simulink model "control_sys_hardware"  (R2024b)
settings: Solver=ode5  StartTime=0.0  StopTime=inf  FixedStep=.0005  RelTol=1e-3
values from neighbouring files (symbols this model uses):
  A = [0, 1, 0, 0, 0, 0, 0, 0, 0 ... (first row only)    [control_sys.m]
  B = [0, 0, 0 ... (first row only)    [control_sys.m]
  b_eq_phi = (n^2)*b_r1 + b_r2 + b_load_phi    (= 46.8203648256)    [control_sys.m]
  b_eq_r = 0.06    [control_sys.m]
  b_eq_theta = (n^2)*b_r1 + b_r2 + b_load_theta    (= 46.8203648256)    [control_sys.m]
  C = [1 0 0 0 0 0 0 0 0 ... (first row only)    [control_sys.m]
  D = [0 0 0 ... (first row only)    [control_sys.m]
  g = 9.81    [control_sys.m]
  J_act_const_phi = (J_act_vert + J_act_horiz)/2    (= 0.17578)    [control_sys.m]
  J_act_const_theta = ((m_act_base + m_act_case + m_act_screw)*(.5588^2) + m_act_rod*(.508^2))/3    (= 0.139191119467)    [control_sys.m]
  J_act_var_phi = (J_act_vert - J_act_horiz)/2    (= -0.17078)    [control_sys.m]
  J_const_phi = J_m1out + J_load_phi    (= 101.81800125)    [control_sys.m]
  J_const_theta = J_m2out    (= 102.01900125)    [control_sys.m]
  J_eq_r = 0.0018    [control_sys.m]
  K = lqr(A,B,Q,R)    [control_sys.m]
  K_r1 = .11    (= 0.11)    [control_sys.m]
  K_r2 = .11    (= 0.11)    [control_sys.m]
  K_r3 = 0.0709    [control_sys.m]
  Kr = inv(C*inv(-A+B*K)*B)    [control_sys.m]
  L_a1 = 0.3    [control_sys.m]
  L_a2 = 0.3    [control_sys.m]
  L_a3 = 0.09    [control_sys.m]
  l_act_const = 0.550    (= 0.55)    [control_sys.m]
  l_act_rod = 0.511175    [control_sys.m]
  m_act = m_act_base + m_act_rod + m_act_screw + m_act_case + m_load    (= 1.364)    [control_sys.m]
  m_act_rod = 0.154    [control_sys.m]
  m_load = 0    [control_sys.m]
  n = 184    [control_sys.m]
  n_3 = 3.07500    (= 3.075)    [control_sys.m]
  p_s = 0.0035    [control_sys.m]
  R_a1 = 1.36    [control_sys.m]
  R_a2 = 1.36    [control_sys.m]
  R_a3 = 2.0500    (= 2.05)    [control_sys.m]
  r_cg_const = (l_act_const*.5*(m_act_case + m_act_screw) + .06*m_act_base)/m_act    (= 0.150795454545)    [control_sys.m]
  tomato_positions = [34; 60; 12.5]    [control_sys.m]
undefined symbols (not defined in the file or in its folder): Continuous, National_Instruments, PCIe, Time
libraries: simulink x15, spsEdgeDetectorLib x15, sldrtlib x13, ctrlSharedLib x1
settings Model: SimulationMode=external  Creator=jcglenn  LastModifiedBy=jcglenn
settings DebuggingCC: UnderSpecifiedDimensionMsg=warning
settings HardwareCC: ProdBitPerLong=64  ProdHWDeviceType=Intel->x86-64 (Linux 64)
settings RTWCC: Description=Simulink Desktop Real-Time  SystemTargetFile=sldrt.tlc  TemplateMakefile=sldrt.tmf  RTWCompilerOptimization=on
settings CodeAppCC: MaxIdLength=95
settings SimulinkDesktopRealTimeCC: TargetLibSuffix=_sldrt.a  TargetPreCompLibLocation=C:\Program Files\MATLAB\R2024b\toolbox\sldrt\lib\win64  ParMdlRefBuildCompliant=on

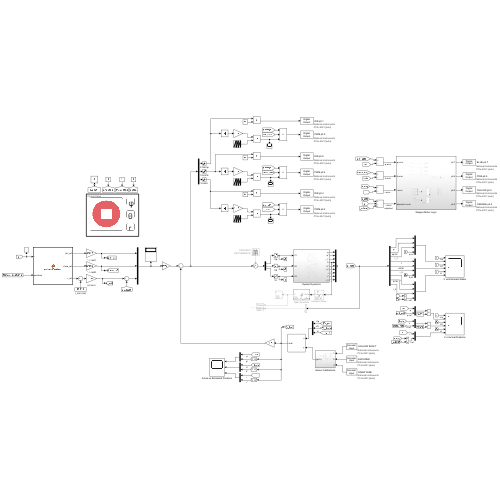
[thumbnail: Simulink's stored preview of the top-level diagram]
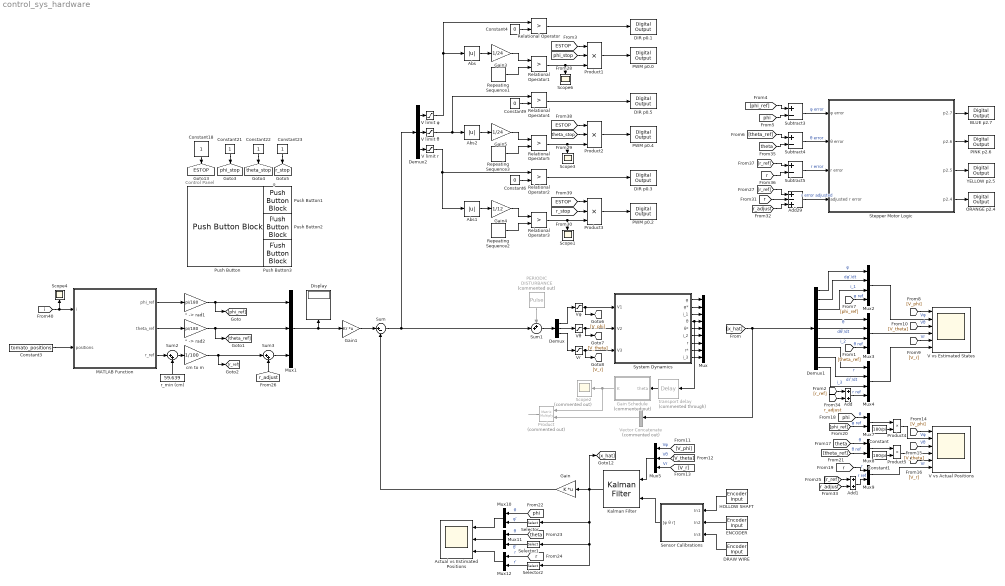
== system control_sys_hardware ==
  note: Control Panel
  note: φ
  note: θ
  note: r
  Abs : Abs  SaturateOnIntegerOverflow=off
  Abs1 : Abs  SaturateOnIntegerOverflow=off
  Abs2 : Abs  SaturateOnIntegerOverflow=off
  Actual vs Estimated Positions : Scope  NumInputPorts=3
  Add : Sum
  Add1 : Sum
  Add29 : Sum  Inputs=+-+
  BLUE p2.7 : sldrtlib/Digital Output  SampleTime=.001  MaxMissedTicks=100  ShowMissedTicks=off  YieldWhenWaiting=off  DrvName=National_Instruments/PCIe-6321  DrvAddress=4294967295  DrvOptions=[0 3 61440 2 0 0 0]  Channels=48  BitMode=1  InitialValue=[]  FinalValue=[]
      settings: AttributesFormatString=National Instruments\nPCIe-6321 [auto]
  Constant : Constant  Value=180/pi
  Constant1 : Constant  Value=180/pi
  Constant{18,21..23} (4 alike) : Constant
  Constant3 : Constant  Value=tomato_positions
  Constant4 : Constant  Value=0
  Constant6 : Constant  Value=0
  Constant9 : Constant  Value=0
  DIR p0.1 : sldrtlib/Digital Output  SampleTime=.001  MaxMissedTicks=100  ShowMissedTicks=off  YieldWhenWaiting=off  DrvName=National_Instruments/PCIe-6321  DrvAddress=4294967295  DrvOptions=[0 63 61440 2 2 2 0]  Channels=2  BitMode=1  InitialValue=[]  FinalValue=[]
      settings: AttributesFormatString=National Instruments\nPCIe-6321 [auto]
  DIR p0.3 : sldrtlib/Digital Output  SampleTime=.001  MaxMissedTicks=100  ShowMissedTicks=off  YieldWhenWaiting=off  DrvName=National_Instruments/PCIe-6321  DrvAddress=4294967295  DrvOptions=[0 63 61440 2 2 2 0]  Channels=4  BitMode=1  InitialValue=[]  FinalValue=[]
      settings: AttributesFormatString=National Instruments\nPCIe-6321 [auto]
  DIR p0.5 : sldrtlib/Digital Output  SampleTime=.001  MaxMissedTicks=100  ShowMissedTicks=off  YieldWhenWaiting=off  DrvName=National_Instruments/PCIe-6321  DrvAddress=4294967295  DrvOptions=[0 63 61440 2 2 2 0]  Channels=6  BitMode=1  InitialValue=[]  FinalValue=[]
      settings: AttributesFormatString=National Instruments\nPCIe-6321 [auto]
  DRAW WIRE : sldrtlib/Encoder Input  SampleTime=.0005  MaxMissedTicks=10  ShowMissedTicks=off  YieldWhenWaiting=off  DrvName=National_Instruments/PCIe-6321  DrvAddress=4294967295  DrvOptions=[0 63 61440 2 2 2 0]  Channels=1  QuadMode=3  IndexPulse=1  InputFilter=Inf  DataType=1
      settings: AttributesFormatString=National Instruments\nPCIe-6321 [auto]
  Demux : Demux  Outputs=3
  Demux1 : Demux  Outputs=9
  Demux2 : Demux  Outputs=3
  Display : Display
  ENCODER : sldrtlib/Encoder Input  SampleTime=.0005  MaxMissedTicks=10  ShowMissedTicks=off  YieldWhenWaiting=off  DrvName=National_Instruments/PCIe-6321  DrvAddress=4294967295  DrvOptions=[0 63 61440 2 2 2 0]  Channels=3  QuadMode=3  IndexPulse=1  InputFilter=Inf  DataType=1
      settings: AttributesFormatString=National Instruments\nPCIe-6321 [auto]
  Gain : Gain  Gain=K  Multiplication=Matrix(K*u)
  Gain Schedule : MATLAB Function  Commented=on  TreatAsAtomicUnit=on
  Gain1 : Gain  Gain=Kr  Multiplication=Matrix(K*u)
  Gain3 : Gain  Gain=1/24
  Gain4 : Gain  Gain=1/12
  Gain5 : Gain  Gain=1/24
  HOLLOW SHAFT : sldrtlib/Encoder Input  SampleTime=.0005  MaxMissedTicks=10  ShowMissedTicks=off  YieldWhenWaiting=off  DrvName=National_Instruments/PCIe-6321  DrvAddress=4294967295  DrvOptions=[0 63 61440 2 2 2 0]  Channels=2  QuadMode=3  IndexPulse=1  InputFilter=Inf  DataType=1
      settings: AttributesFormatString=National Instruments\nPCIe-6321 [auto]
  Kalman Filter : ctrlSharedLib/Kalman Filter  TimeDomain=Continuous-Time  UseCurrentEstimator=on  ModelSource=Individual A, B, C, D matrices  ModelSourceVariable=ss(0.95,1,1,0,1)  A=A  B=B  C=C  D=D  NumberOfStates=1  NumberOfInputs=1  NumberOfOutputs=1  InitialEstimateSource=Dialog  X0=[0; 0; 0; 0; 0; 0; 0; 0; 0]  P0=10  UseK=off  UseGH=off  NumberOfProcessNoiseInputs=1  G=1  TimeInvariantG=on  H=0  TimeInvariantH=on  Q=1  TimeInvariantQ=on  R=1  TimeInvariantR=on  N=0  TimeInvariantN=on  AddInputPort=on  AddEnablePort=off  OutputEstimatedY=off  OutputP=off  Ts=-1
  MATLAB Function : MATLAB Function  TreatAsAtomicUnit=on
  Mux : Mux  Inputs=9
  Mux1 : Mux  Inputs=3
  Mux{7..12} (6 alike) : Mux  Inputs=2
  Mux2 : Mux
  Mux3 : Mux
  Mux4 : Mux
  Mux5 : Mux  Inputs=3
  ORANGE p2.4 : sldrtlib/Digital Output  SampleTime=.001  MaxMissedTicks=100  ShowMissedTicks=off  YieldWhenWaiting=off  DrvName=National_Instruments/PCIe-6321  DrvAddress=4294967295  DrvOptions=[0 3 61440 2 0 0 0]  Channels=45  BitMode=1  InitialValue=[]  FinalValue=[]
      settings: AttributesFormatString=National Instruments\nPCIe-6321 [auto]
  PERIODIC DISTURBANCE : DiscretePulseGenerator  Commented=on  PulseType=Time based  Amplitude=3  Period=15  PulseWidth=5  PhaseDelay=5
  PINK p2.6 : sldrtlib/Digital Output  SampleTime=.001  MaxMissedTicks=100  ShowMissedTicks=off  YieldWhenWaiting=off  DrvName=National_Instruments/PCIe-6321  DrvAddress=4294967295  DrvOptions=[0 3 61440 2 0 0 0]  Channels=47  BitMode=1  InitialValue=[]  FinalValue=[]
      settings: AttributesFormatString=National Instruments\nPCIe-6321 [auto]
  PWM p0.0 : sldrtlib/Digital Output  SampleTime=0.001  MaxMissedTicks=100  ShowMissedTicks=off  YieldWhenWaiting=off  DrvName=National_Instruments/PCIe-6321  DrvAddress=4294967295  DrvOptions=[0 63 61440 2 2 2 0]  Channels=1  BitMode=1  InitialValue=[]  FinalValue=[]
      settings: AttributesFormatString=National Instruments\nPCIe-6321 [auto]
  PWM p0.2 : sldrtlib/Digital Output  SampleTime=0.001  MaxMissedTicks=100  ShowMissedTicks=off  YieldWhenWaiting=off  DrvName=National_Instruments/PCIe-6321  DrvAddress=4294967295  DrvOptions=[0 63 61440 2 2 2 0]  Channels=3  BitMode=1  InitialValue=[]  FinalValue=[]
      settings: AttributesFormatString=National Instruments\nPCIe-6321 [auto]
  PWM p0.4 : sldrtlib/Digital Output  SampleTime=0.001  MaxMissedTicks=100  ShowMissedTicks=off  YieldWhenWaiting=off  DrvName=National_Instruments/PCIe-6321  DrvAddress=4294967295  DrvOptions=[0 63 61440 2 2 2 0]  Channels=5  BitMode=1  InitialValue=[]  FinalValue=[]
      settings: AttributesFormatString=National Instruments\nPCIe-6321 [auto]
  Product : Product  Commented=on  Multiplication=Matrix(*)
  Product1 : Product  Inputs=3
  Product2 : Product  Inputs=3
  Product3 : Product  Inputs=3
  Product4 : Product
  Product5 : Product
  Push Button{,1..3} (4 alike) : PushButtonBlock  ButtonText=‎  OnValue=0  Opacity=.35  ButtonType=Latch  OffValue=1.000000
  Relational Operator{,1..5} (6 alike) : RelationalOperator  Operator=>  OutDataTypeStr=boolean  RndMeth=Simplest  InputSameDT=off
  Repeating Sequence1 : simulink/Sources/Repeating Sequence  rep_seq_t=[0 .005]  rep_seq_y=[.005 1]
  Repeating Sequence2 : simulink/Sources/Repeating Sequence  rep_seq_t=[0 .005]  rep_seq_y=[.005 1]
  Repeating Sequence3 : simulink/Sources/Repeating Sequence  rep_seq_t=[0 .005]  rep_seq_y=[.005 1]
  Scope{1,3..4,6} (4 alike) : Scope
  Scope2 : Scope  Commented=on
  Selector : Selector  InputPortWidth=9  IndexOptions=Index vector (dialog)  Indices=[1]  OutputSizes=1
  Selector1 : Selector  InputPortWidth=9  IndexOptions=Index vector (dialog)  Indices=[4]  OutputSizes=1
  Selector2 : Selector  InputPortWidth=9  IndexOptions=Index vector (dialog)  Indices=[7]  OutputSizes=1
  Sensor Calibrations : Subsystem
  Stepper Motor Logic : Subsystem
  Subtract3 : Sum  Inputs=+-
  Subtract4 : Sum  Inputs=+-
  Subtract5 : Sum  Inputs=+-
  Sum : Sum  Inputs=|+-
  Sum1 : Sum  Inputs=++|
  Sum2 : Sum  Inputs=|++
  Sum3 : Sum  Inputs=|++
  System Dynamics : Subsystem
  V limit r : Saturate  UpperLimit=12  LowerLimit=-12
  V limit θ : Saturate  UpperLimit=24  LowerLimit=-24
  V limit φ : Saturate  UpperLimit=24  LowerLimit=-24
  V vs Actual Positions : Scope  NumInputPorts=6
  V vs Estimated States : Scope  NumInputPorts=6
  Vector Concatenate : Concatenate  Commented=on  NumInputs=1  Mode=Multidimensional array
  Vr : Saturate  UpperLimit=12  LowerLimit=-12
  Vθ : Saturate  UpperLimit=24  LowerLimit=-24
  Vφ : Saturate  UpperLimit=24  LowerLimit=-24
  YELLOW p2.5 : sldrtlib/Digital Output  SampleTime=.001  MaxMissedTicks=100  ShowMissedTicks=off  YieldWhenWaiting=off  DrvName=National_Instruments/PCIe-6321  DrvAddress=4294967295  DrvOptions=[0 3 61440 2 0 0 0]  Channels=46  BitMode=1  InitialValue=[]  FinalValue=[]
      settings: AttributesFormatString=National Instruments\nPCIe-6321 [auto]
  cm to m : Gain  Gain=1/100
  r_min (cm) : Constant  Value=59.639
  transport delay : TransportDelay  Commented=through  DelayTime=.1
  "° -> rad1" : Gain  Gain=pi/180
  "° -> rad2" : Gain  Gain=pi/180
  tag scope: ESTOP=global, phi_stop=global, r_stop=global, theta_stop=global
  wires:
  MATLAB Function/1(phi_ref) -> "° -> rad1"/1
  MATLAB Function/2(theta_ref) -> "° -> rad2"/1
  System Dynamics/4(θ) -> transport delay/1, Mux/4
  "° -> rad1"/1 -> Mux1/1, [phi_ref]
  "° -> rad2"/1 -> Mux1/2, [theta_ref]
  Gain1/1 -> Sum/1
  Product/1 -> ?
  Demux/1 -> Vφ/1
  Demux/2 -> Vθ/1
  Mux1/1 -> Display/1, Gain1/1
  Sum/1 -> Sum1/2, Demux2/1
  PERIODIC DISTURBANCE/1 -> Sum1/1
  Demux1/4 -> Mux3/1  "θ"
  Demux1/1 -> Mux2/1  "φ"
  Gain Schedule/1(K) -> Product/1, Scope2/1
  Vector Concatenate/1 -> Product/2
  Sum1/1 -> Demux/1
  transport delay/1 -> Gain Schedule/1(theta)
  System Dynamics/1(φ) -> Mux/1
  System Dynamics/2(φ*) -> Mux/2
  System Dynamics/3(i_1) -> Mux/3
  System Dynamics/5(θ*) -> Mux/5
  System Dynamics/6(i_2) -> Mux/6
  System Dynamics/7(r) -> Mux/7
  System Dynamics/8(r*) -> Mux/8
  System Dynamics/9(i_3) -> Mux/9
  MATLAB Function/3(r_ref) -> Sum2/1
  cm to m/1 -> Sum3/1, [r_ref]
  Demux/3 -> Vr/1
  Demux1/7 -> Mux4/1  "r"
  Demux1/3 -> Mux2/3  "i_1"
  Demux1/2 -> Mux2/2  "dφ ̂/dt"
  Demux1/5 -> Mux3/2  "dθ ̂/dt"
  Demux1/6 -> Mux3/3  "i_2"
  Demux1/8 -> Mux4/2  "dr ̂/dt"
  Demux1/9 -> Mux4/3  "i_3"
  [theta_ref] -> Mux3/4  "θ ref"
  Abs/1 -> Gain3/1
  Repeating Sequence1/1 -> Relational Operator1/2
  Relational Operator1/1 -> Scope6/1, Product1/3
  Constant4/1 -> Relational Operator/2
  Product1/1 -> PWM p0.0/1
  Gain3/1 -> Relational Operator1/1
  Demux2/1 -> V limit φ/1
  Relational Operator/1 -> DIR p0.1/1
  Gain4/1 -> Relational Operator3/1
  Demux2/3 -> V limit r/1
  Relational Operator2/1 -> DIR p0.3/1
  Constant6/1 -> Relational Operator2/2
  Relational Operator3/1 -> Scope1/1, Product3/3
  Repeating Sequence2/1 -> Relational Operator3/2
  Abs1/1 -> Gain4/1
  Product3/1 -> PWM p0.2/1
  Constant9/1 -> Relational Operator4/2
  Repeating Sequence3/1 -> Relational Operator5/2
  Relational Operator5/1 -> Product2/3, Scope3/1
  Relational Operator4/1 -> DIR p0.5/1
  Demux2/2 -> V limit θ/1
  Abs2/1 -> Gain5/1
  Product2/1 -> PWM p0.4/1
  Gain5/1 -> Relational Operator5/1
  Gain/1 -> Sum/2
  V limit θ/1 -> Relational Operator4/1, Abs2/1
  V limit r/1 -> Relational Operator2/1, Abs1/1
  V limit φ/1 -> Abs/1, Relational Operator/1
  Vφ/1 -> System Dynamics/1(V1), [V_phi]
  Vθ/1 -> [V_theta], System Dynamics/2(V2)
  Vr/1 -> [V_r], System Dynamics/3(V3)
  Sum2/1 -> cm to m/1
  r_min (cm)/1 -> Sum2/2
  [phi_ref] -> Mux2/4  "φ ref"
  [V_r] -> V vs Estimated States/5  "Vr"
  [V_theta] -> V vs Estimated States/3  "Vθ"
  [V_phi] -> V vs Estimated States/1  "Vφ"
  Mux3/1 -> V vs Estimated States/4
  Mux2/1 -> V vs Estimated States/2
  Mux4/1 -> V vs Estimated States/6
  Mux5/1 -> Kalman Filter/1
  [V_phi] -> Mux5/1  "Vφ"
  [V_theta] -> Mux5/2  "Vθ"
  [V_r] -> Mux5/3  "Vr"
  [V_phi] -> V vs Actual Positions/1  "Vφ"
  [V_theta] -> V vs Actual Positions/3  "Vθ"
  [V_r] -> V vs Actual Positions/5  "Vr"
  [phi] -> Mux7/1  "φ"
  [theta] -> Mux8/1  "θ"
  [phi_ref] -> Mux7/2  "φ ref"
  [theta_ref] -> Mux8/2  "θ ref"
  [x_hat] -> Demux1/1, Vector Concatenate/1
  Kalman Filter/1 -> Selector2/1, Selector1/1, Selector/1, Gain/1, [x_hat]
  Mux10/1 -> Actual vs Estimated Positions/1
  Mux11/1 -> Actual vs Estimated Positions/2
  Mux12/1 -> Actual vs Estimated Positions/3
  [phi] -> Mux10/1  "φ"
  [theta] -> Mux11/1  "θ"
  [r] -> Mux12/1  "r"
  Selector/1 -> Mux10/2  "φ ̂"
  Selector1/1 -> Mux11/2  "θ ̂"
  Selector2/1 -> Mux12/2  "r ̂"
  Mux7/1 -> Product4/1
  Constant18/1 -> [ESTOP]
  [phi_stop] -> Product1/2
  HOLLOW SHAFT/1 -> Sensor Calibrations/1(In1)
  ENCODER/1 -> Sensor Calibrations/2(In2)
  DRAW WIRE/1 -> Sensor Calibrations/3(In3)
  Sensor Calibrations/1("[φ θ r]") -> Kalman Filter/2
  [r_ref] -> Subtract5/1
  [theta_ref] -> Subtract4/1
  [r] -> Subtract5/2
  [phi_ref] -> Subtract3/1
  [theta] -> Subtract4/2
  [phi] -> Subtract3/2
  Subtract3/1 -> Stepper Motor Logic/1(φ error)  "φ error"
  Subtract4/1 -> Stepper Motor Logic/2(θ error)  "θ error"
  Subtract5/1 -> Stepper Motor Logic/3(r error)  "r error"
  Stepper Motor Logic/1(p2.7) -> BLUE p2.7/1
  Stepper Motor Logic/2(p2.6) -> PINK p2.6/1
  Stepper Motor Logic/3(p2.5) -> YELLOW p2.5/1
  Stepper Motor Logic/4(p2.4) -> ORANGE p2.4/1
  Constant21/1 -> [phi_stop]
  Constant22/1 -> [theta_stop]
  Constant23/1 -> [r_stop]
  [ESTOP] -> Product1/1
  [theta_stop] -> Product2/2
  [ESTOP] -> Product2/1
  [r_stop] -> Product3/2
  [ESTOP] -> Product3/1
  Sum3/1 -> Mux1/3
  [r_adjust] -> Sum3/2
  Add29/1 -> Stepper Motor Logic/4(adjusted r error)  "r error adjusted"
  [r_ref] -> Add29/1
  [r] -> Add29/2
  [r_adjust] -> Add29/3
  Product4/1 -> V vs Actual Positions/2
  Constant/1 -> Product4/2
  Mux9/1 -> V vs Actual Positions/6
  Constant1/1 -> Product5/2
  Mux8/1 -> Product5/1
  Product5/1 -> V vs Actual Positions/4
  [r] -> Mux9/1  "r"
  [r_ref] -> Add1/1
  [r_adjust] -> Add1/2
  Add1/1 -> Mux9/2  "r ref"
  [r_ref] -> Add/1
  [r_adjust] -> Add/2
  Add/1 -> Mux4/4  "r ref"
  [i] -> MATLAB Function/1(i), Scope4/1
  Constant3/1 -> MATLAB Function/2(positions)

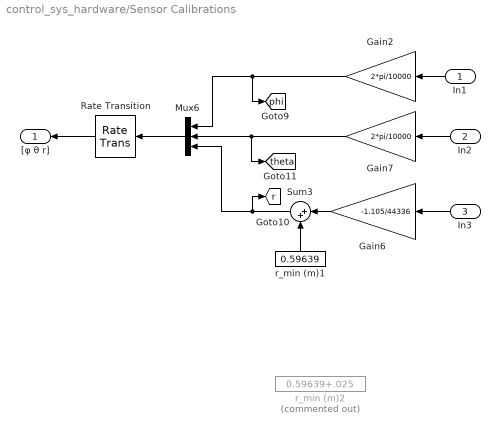
== system control_sys_hardware/Sensor Calibrations ==
  In1 : Inport
  In2 : Inport  Port=2
  In3 : Inport  Port=3
  Gain2 : Gain  Gain=2*pi/10000
  Gain6 : Gain  Gain=-1.105/44336
  Gain7 : Gain  Gain=2*pi/10000
  Mux6 : Mux  Inputs=3
  Rate Transition : RateTransition
  Sum3 : Sum  Inputs=|++
  r_min (m)1 : Constant  Value=0.59639
  r_min (m)2 : Constant  Commented=on  Value=0.59639+.025
  "[φ θ r]" : Outport
  tag scope: phi=global, r=global, theta=global
  wires:
  Sum3/1 -> Mux6/3, [r]
  Mux6/1 -> Rate Transition/1
  Gain2/1 -> [phi], Mux6/1
  r_min (m)1/1 -> Sum3/2
  Gain7/1 -> [theta], Mux6/2
  Gain6/1 -> Sum3/1
  In2/1 -> Gain7/1
  In1/1 -> Gain2/1
  In3/1 -> Gain6/1
  Rate Transition/1 -> "[φ θ r]"/1

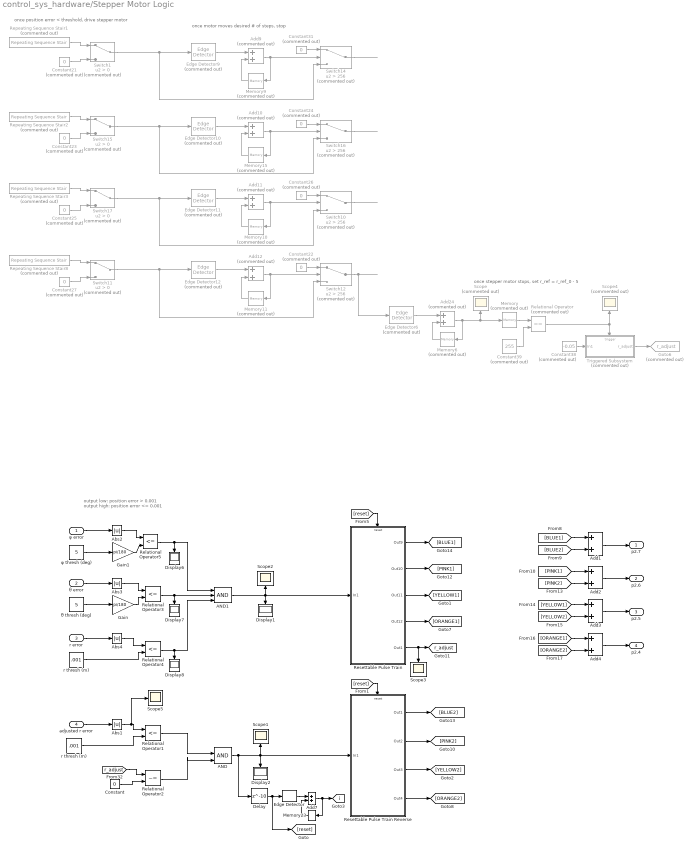
== system control_sys_hardware/Stepper Motor Logic ==
  note: once stepper motor stops, set r_ref = r_ref_0 - 5
  note: once motor moves desired # of steps, stop
  note: once position error < threshold, drive stepper motor
  note: output low: position error > 0.001
      | output high: position error <= 0.001
  φ error : Inport
  θ error : Inport  Port=2
  r error : Inport  Port=3
  adjusted r error : Inport  Port=4
  AND : Logic  IconShape=distinctive  AllPortsSameDT=off  OutDataTypeStr=boolean
  AND1 : Logic  Inputs=3  IconShape=distinctive  AllPortsSameDT=off  OutDataTypeStr=boolean
  Abs{1..4} (4 alike) : Abs  SaturateOnIntegerOverflow=off
  Add{1..4} (4 alike) : Sum
  Add{9..12,24} (5 alike) : Sum  Commented=on  OutDataTypeStr=double  AccumDataTypeStr=double
  Add7 : Sum  OutDataTypeStr=double  AccumDataTypeStr=double
  Constant : Constant  Value=0
  Constant{21..27,31} (8 alike) : Constant  Commented=on  Value=0
  Constant38 : Constant  Commented=on  Value=-0.05
  Constant39 : Constant  Commented=on  Value=255
  Delay : Delay  DelayLength=10  SampleTime=1
  Display{1..2,6..8} (5 alike) : Display
  Edge Detector : spsEdgeDetectorLib/Edge Detector  model=Rising  ic=0  Ts=0
      settings: LibrarySourceBlock=sps_lib/Control/Edge Detector
  Edge Detector{6,9..12} (5 alike) : spsEdgeDetectorLib/Edge Detector  Commented=on  model=Rising  ic=0  Ts=0
      settings: LibrarySourceBlock=sps_lib/Control/Edge Detector
  Gain : Gain  Gain=pi/180
  Gain1 : Gain  Gain=pi/180
  Goto6 : Goto  Commented=on  GotoTag=r_adjust  TagVisibility=global
  Memory : Memory  Commented=on
  Memory{6,9..11,15} (5 alike) : Memory  Commented=on  InheritSampleTime=on
  Memory23 : Memory  InitialCondition=1  InheritSampleTime=on
  Relational Operator : RelationalOperator  Commented=on  Operator===  OutDataTypeStr=boolean  RndMeth=Simplest  InputSameDT=off
  Relational Operator{1,3..5} (4 alike) : RelationalOperator  Operator=<=  OutDataTypeStr=boolean  RndMeth=Simplest  InputSameDT=off
  Relational Operator2 : RelationalOperator  Operator=~=  OutDataTypeStr=boolean  RndMeth=Simplest  InputSameDT=off
  Repeating Sequence Stair1 : simulink/Sources/Repeating Sequence Stair  Commented=on  OutValues=[1 0 0 0].'  tsamp=.01  OutMin=[]  OutMax=[]  OutDataTypeStr=double  OutputDataTypeScalingMode=double  OutDataType=fixdt(0,8)  ConRadixGroup=Best Precision: Vector-wise  OutScaling=2^-12
  Repeating Sequence Stair2 : simulink/Sources/Repeating Sequence Stair  Commented=on  OutValues=[0 1 0 0].'  tsamp=.01  OutMin=[]  OutMax=[]  OutDataTypeStr=double  OutputDataTypeScalingMode=double  OutDataType=fixdt(0,8)  ConRadixGroup=Best Precision: Vector-wise  OutScaling=2^-12
  Repeating Sequence Stair3 : simulink/Sources/Repeating Sequence Stair  Commented=on  OutValues=[0 0 1 0].'  tsamp=.01  OutMin=[]  OutMax=[]  OutDataTypeStr=double  OutputDataTypeScalingMode=double  OutDataType=fixdt(0,8)  ConRadixGroup=Best Precision: Vector-wise  OutScaling=2^-12
  Repeating Sequence Stair8 : simulink/Sources/Repeating Sequence Stair  Commented=on  OutValues=[0 0 0 1].'  tsamp=.01  OutMin=[]  OutMax=[]  OutDataTypeStr=double  OutputDataTypeScalingMode=double  OutDataType=fixdt(0,8)  ConRadixGroup=Best Precision: Vector-wise  OutScaling=2^-12
  Resettable Pulse Train : Subsystem  TreatAsAtomicUnit=on
  Resettable Pulse Train Reverse : Subsystem  TreatAsAtomicUnit=on
  Scope : Scope  Commented=on
  Scope{1..3,5} (4 alike) : Scope
  Scope4 : Scope  Commented=on
  Switch{1,11,15,17} (4 alike) : Switch  Commented=on  Criteria=u2 > Threshold  SaturateOnIntegerOverflow=off  InputSameDT=off
  Switch{10,12,14,16} (4 alike) : Switch  Commented=on  Criteria=u2 > Threshold  Threshold=256  SaturateOnIntegerOverflow=off  InputSameDT=off
  Triggered Subsystem : Subsystem  Commented=on  TreatAsAtomicUnit=on
  r thresh (m) : Constant  Value=.001
  "r thresh (m) " : Constant  Value=.001
  θ thresh (deg) : Constant  Value=5
  φ thresh (deg) : Constant  Value=5
  p2.7 : Outport
  p2.6 : Outport  Port=2
  p2.5 : Outport  Port=3
  p2.4 : Outport  Port=4
  tag scope: i=global, r_adjust=global
  wires:
  Constant26/1 -> Switch10/1
  Relational Operator4/1 -> Display8/1, AND1/3
  Switch17/1 -> Switch10/3, Edge Detector11/1
  Memory15/1 -> Add10/2
  Edge Detector10/1 -> Add10/1
  Add9/1 -> Switch14/2, Memory9/1
  Memory10/1 -> Add11/2
  Constant23/1 -> Switch15/3
  Switch16/1 -> ?
  Edge Detector11/1 -> Add11/1
  Switch1/1 -> Switch14/3, Edge Detector9/1
  Add10/1 -> Switch16/2, Memory15/1
  Constant27/1 -> Switch11/3
  Add12/1 -> Switch12/2, Memory11/1
  Repeating Sequence Stair3/1 -> Switch17/1
  Relational Operator5/1 -> Display6/1, AND1/1
  Switch11/1 -> Switch12/3, Edge Detector12/1
  Constant24/1 -> Switch16/1
  Add11/1 -> Switch10/2, Memory10/1
  Repeating Sequence Stair1/1 -> Switch1/1
  Switch14/1 -> ?
  Constant22/1 -> Switch12/1
  Memory11/1 -> Add12/2
  Repeating Sequence Stair8/1 -> Switch11/1
  Switch15/1 -> Switch16/3, Edge Detector10/1
  Memory9/1 -> Add9/2
  Repeating Sequence Stair2/1 -> Switch15/1
  Constant25/1 -> Switch17/3
  Edge Detector12/1 -> Add12/1
  Edge Detector9/1 -> Add9/1
  Constant21/1 -> Switch1/3
  Switch10/1 -> ?
  Relational Operator3/1 -> Display7/1, AND1/2
  Constant31/1 -> Switch14/1
  Memory/1 -> Relational Operator/1
  Edge Detector6/1 -> Add24/1
  Triggered Subsystem/1(r_adjust) -> Goto6/1
  Memory6/1 -> Add24/2
  Switch12/1 -> Edge Detector6/1
  Add24/1 -> Memory/1, Scope/1, Memory6/1
  Relational Operator/1 -> Scope4/1, Triggered Subsystem/Trigger
  Constant38/1 -> Triggered Subsystem/1(In1)
  Constant39/1 -> Relational Operator/2
  Resettable Pulse Train/3(Out11) -> [YELLOW1]
  Resettable Pulse Train/2(Out10) -> [PINK1]
  Resettable Pulse Train/4(Out12) -> [ORANGE1]
  Resettable Pulse Train/1(Out9) -> [BLUE1]
  Resettable Pulse Train/5(Out1) -> [r_adjust], Scope3/1
  [reset] -> Resettable Pulse Train/Reset
  AND1/1 -> Display1/1, Scope2/1, Resettable Pulse Train/1(In1)
  [YELLOW2] -> Add3/2
  [ORANGE2] -> Add4/2
  [PINK1] -> Add2/1
  [ORANGE1] -> Add4/1
  Add3/1 -> p2.5/1
  [YELLOW1] -> Add3/1
  [BLUE2] -> Add1/2
  [BLUE1] -> Add1/1
  Add1/1 -> p2.7/1
  Add2/1 -> p2.6/1
  [PINK2] -> Add2/2
  Add4/1 -> p2.4/1
  adjusted r error/1 -> Abs1/1
  Abs1/1 -> Scope5/1, Relational Operator1/1
  "r thresh (m) "/1 -> Relational Operator1/2
  Relational Operator1/1 -> AND/1
  [r_adjust] -> Relational Operator2/1
  Constant/1 -> Relational Operator2/2
  Relational Operator2/1 -> AND/2
  AND/1 -> Delay/1, Resettable Pulse Train Reverse/1(In1), Scope1/1, Display2/1
  Resettable Pulse Train Reverse/4(Out4) -> [ORANGE2]
  Resettable Pulse Train Reverse/2(Out2) -> [PINK2]
  Resettable Pulse Train Reverse/3(Out3) -> [YELLOW2]
  [reset] -> Resettable Pulse Train Reverse/Reset
  Resettable Pulse Train Reverse/1(Out1) -> [BLUE2]
  Abs4/1 -> Relational Operator4/1
  Gain1/1 -> Relational Operator5/2
  r error/1 -> Abs4/1
  Gain/1 -> Relational Operator3/2
  φ thresh (deg)/1 -> Gain1/1
  θ error/1 -> Abs3/1
  φ error/1 -> Abs2/1
  Abs3/1 -> Relational Operator3/1
  θ thresh (deg)/1 -> Gain/1
  r thresh (m)/1 -> Relational Operator4/2
  Abs2/1 -> Relational Operator5/1
  Edge Detector/1 -> Add7/1
  Add7/1 -> [i], Memory23/1
  Memory23/1 -> Add7/2
  Delay/1 -> [reset], Edge Detector/1

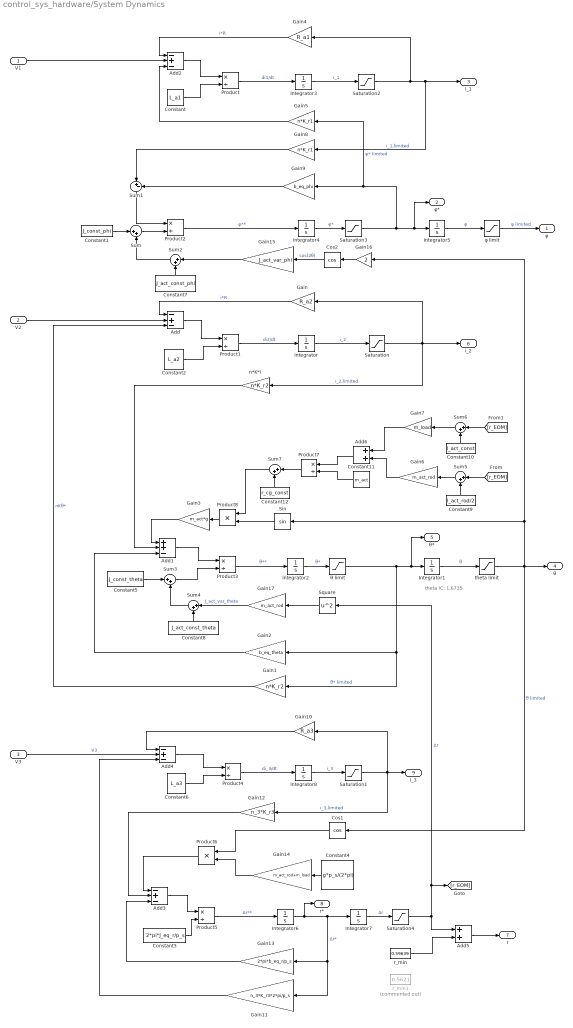
== system control_sys_hardware/System Dynamics ==
  note: theta IC: 1.6735
  V1 : Inport
  V2 : Inport  Port=2
  V3 : Inport  Port=3
  Add{,2..4} (4 alike) : Sum  Inputs=-+-
  Add1 : Sum  Inputs=++-
  Add5 : Sum
  Add6 : Sum
  Constant : Constant  Value=L_a1
  Constant1 : Constant  Value=J_const_phi
  Constant10 : Constant  Value=l_act_const
  Constant11 : Constant  Value=m_act
  Constant12 : Constant  Value=r_cg_const
  Constant2 : Constant  Value=L_a2
  Constant3 : Constant  Value=2*pi*J_eq_r/p_s
  Constant4 : Constant  Value=g*p_s/(2*pi)
  Constant5 : Constant  Value=J_const_theta
  Constant6 : Constant  Value=L_a3
  Constant7 : Constant  Value=J_act_const_phi
  Constant8 : Constant  Value=J_act_const_theta
  Constant9 : Constant  Value=l_act_rod/2
  Cos1 : Trigonometry  Operator=cos
  Cos2 : Trigonometry  Operator=cos
  Gain : Gain  Gain=R_a2
  Gain1 : Gain  Gain=n*K_r2
  Gain10 : Gain  Gain=R_a3
  Gain11 : Gain  Gain=n_3*K_r3*2*pi/p_s
  Gain12 : Gain  Gain=n_3*K_r3
  Gain13 : Gain  Gain=2*pi*b_eq_r/p_s
  Gain14 : Gain  Gain=m_act_rod+m_load
  Gain15 : Gain  Gain=J_act_var_phi
  Gain16 : Gain  Gain=2
  Gain17 : Gain  Gain=m_act_rod
  Gain2 : Gain  Gain=b_eq_theta
  Gain3 : Gain  Gain=m_act*g
  Gain4 : Gain  Gain=R_a1
  Gain5 : Gain  Gain=n*K_r1
  Gain6 : Gain  Gain=m_act_rod
  Gain7 : Gain  Gain=m_load
  Gain8 : Gain  Gain=n*K_r1
  Gain9 : Gain  Gain=b_eq_phi
  Integrator{,1..8} (9 alike) : Integrator
  Product{,1..5,7} (7 alike) : Product  Inputs=*/
  Product6 : Product
  Product8 : Product
  Saturation : Saturate  UpperLimit=6.5  LowerLimit=-6.5
  Saturation1 : Saturate  UpperLimit=5  LowerLimit=-5
  Saturation2 : Saturate  UpperLimit=6.5  LowerLimit=-6.5
  Saturation3 : Saturate  UpperLimit=1.25  LowerLimit=-1.25
  Saturation4 : Saturate  UpperLimit=.4572  LowerLimit=0
  Sin : Trigonometry
  Square : Math  Operator=square
  Sum{,2..7} (7 alike) : Sum  Inputs=|++
  Sum1 : Sum  Inputs=|+-
  n*K*i : Gain  Gain=n*K_r2
  r_min : Constant  Value=0.59639
  r_min1 : Constant  Commented=on  Value=0.5621
  theta limit : Saturate  UpperLimit=1.6735  LowerLimit=-pi/4
  θ limit : Saturate  UpperLimit=1.25  LowerLimit=-1.25
  φ limit : Saturate  UpperLimit=pi  LowerLimit=-pi
  φ : Outport
  φ* : Outport  Port=2
  i_1 : Outport  Port=3
  θ : Outport  Port=4
  θ* : Outport  Port=5
  i_2 : Outport  Port=6
  r : Outport  Port=7
  r* : Outport  Port=8
  i_3 : Outport  Port=9
  wires:
  V1/1 -> Add2/2
  V2/1 -> Add/2
  Integrator7/1 -> Saturation4/1  "Δr"
  Gain14/1 -> Product6/2
  Constant4/1 -> Gain14/1
  Cos1/1 -> Product6/1
  V3/1 -> Add4/2  "V3"
  Product6/1 -> Add3/1
  Saturation1/1 -> i_3/1, Gain10/1, Gain12/1  "i_3,limited"
  Integrator/1 -> Saturation/1  "i_2"
  Constant6/1 -> Product4/2
  theta limit/1 -> Gain16/1, Sin/1, Cos1/1, θ/1  "θ limited"
  Gain9/1 -> Sum1/2
  Sin/1 -> Product8/2
  Gain1/1 -> Add/3  "nKθ*"
  Add1/1 -> Product3/1
  Gain12/1 -> Add3/2
  Gain3/1 -> Add1/1
  Integrator2/1 -> θ limit/1  "θ*"
  Integrator4/1 -> Saturation3/1  "φ*"
  n*K*i/1 -> Add1/2
  Gain10/1 -> Add4/1
  Sum/1 -> Product2/2
  Gain2/1 -> Add1/3
  Constant3/1 -> Product5/2
  Saturation2/1 -> Gain4/1, i_1/1, Gain8/1  "i_1,limited"
  Add3/1 -> Product5/1
  Product5/1 -> Integrator6/1  "Δr**"
  Product1/1 -> Integrator/1  "di2/dt"
  Product3/1 -> Integrator2/1  "θ**"
  Add4/1 -> Product4/1
  Gain/1 -> Add/1  "i*R"
  Integrator6/1 -> r*/1, Gain13/1, Gain11/1, Integrator7/1  "Δr*"
  Add2/1 -> Product/1
  Product4/1 -> Integrator8/1  "di_3/dt"
  Product/1 -> Integrator3/1  "di1/dt"
  Constant5/1 -> Sum3/1
  Sum1/1 -> Product2/1
  Gain5/1 -> Add2/3
  Integrator8/1 -> Saturation1/1  "i_3"
  Constant1/1 -> Sum/1
  Product2/1 -> Integrator4/1  "φ**"
  φ limit/1 -> φ/1  "φ limited"
  Add/1 -> Product1/1
  Saturation/1 -> n*K*i/1, i_2/1, Gain/1  "i_2,limited"
  Gain11/1 -> Add4/3
  Integrator3/1 -> Saturation2/1  "i_1"
  θ limit/1 -> Gain1/1, Gain2/1, θ*/1, Integrator1/1  "θ* limited"
  Gain8/1 -> Sum1/1
  Integrator5/1 -> φ limit/1  "φ"
  Constant/1 -> Product/2
  Saturation3/1 -> Gain9/1, Gain5/1, φ*/1, Integrator5/1  "φ* limited"
  Gain13/1 -> Add3/3
  Gain4/1 -> Add2/1  "i*R"
  Constant2/1 -> Product1/2
  Sum2/1 -> Sum/2
  Integrator1/1 -> theta limit/1  "θ"
  Saturation4/1 -> Add5/1, [r_EOM], Square/1  "Δr"
  r_min/1 -> Add5/2
  Add5/1 -> r/1
  Gain15/1 -> Sum2/1
  Gain16/1 -> Cos2/1
  Constant7/1 -> Sum2/2
  Cos2/1 -> Gain15/1  "cos(2θ)"
  Sum3/1 -> Product3/2
  Sum4/1 -> Sum3/2
  Constant8/1 -> Sum4/2
  Gain17/1 -> Sum4/1  "J_act_var_theta"
  [r_EOM] -> Sum5/1
  Constant9/1 -> Sum5/2
  Sum5/1 -> Gain6/1
  Gain6/1 -> Add6/2
  Constant10/1 -> Sum6/2
  [r_EOM] -> Sum6/1
  Sum6/1 -> Gain7/1
  Gain7/1 -> Add6/1
  Add6/1 -> Product7/1
  Constant11/1 -> Product7/2
  Product7/1 -> Sum7/1
  Constant12/1 -> Sum7/2
  Square/1 -> Gain17/1
  Product8/1 -> Gain3/1
  Sum7/1 -> Product8/1

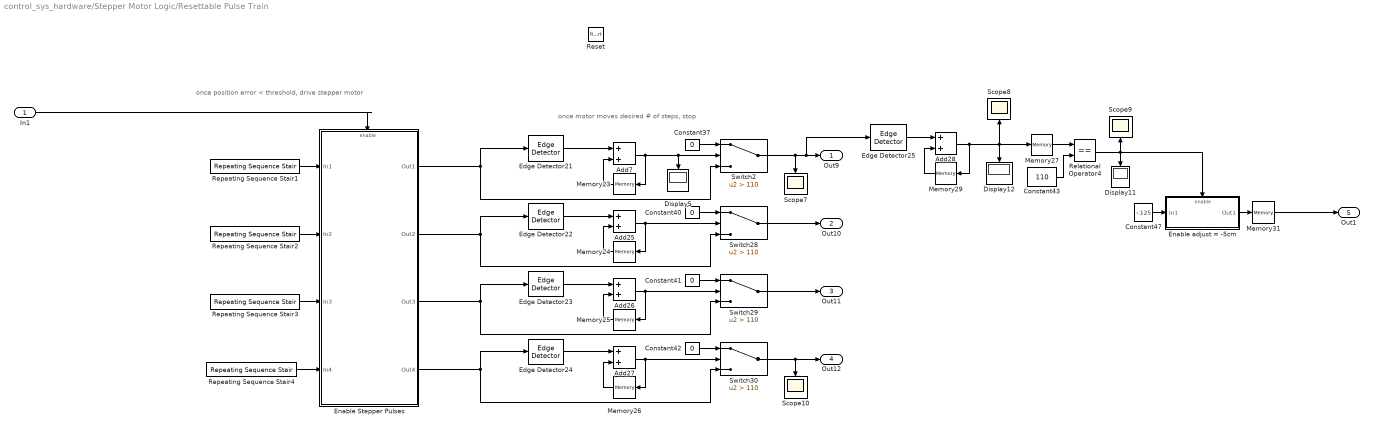
== system control_sys_hardware/Stepper Motor Logic/Resettable Pulse Train ==
  note: once motor moves desired # of steps, stop
  note: once position error < threshold, drive stepper motor
  In1 : Inport
  Reset : ResetPort  DisableCoverage=on
  Add{7,25..28} (5 alike) : Sum  OutDataTypeStr=double  AccumDataTypeStr=double
  Constant{37,40..42} (4 alike) : Constant  Value=0
  Constant43 : Constant  Value=110
  Constant47 : Constant  Value=-.125
  Display11 : Display
  Display12 : Display
  Display5 : Display
  Edge Detector{21..25} (5 alike) : spsEdgeDetectorLib/Edge Detector  model=Rising  ic=0  Ts=0
  Enable Stepper Pulses : Subsystem  TreatAsAtomicUnit=on
  Enable adjust = -5cm : Subsystem  TreatAsAtomicUnit=on
  Memory{23..27,29,31} (7 alike) : Memory  InheritSampleTime=on
  Relational Operator4 : RelationalOperator  Operator===  OutDataTypeStr=boolean  RndMeth=Simplest  InputSameDT=off
  Repeating Sequence Stair1 : simulink/Sources/Repeating Sequence Stair  OutValues=[0 0 0 1].'  tsamp=.01  OutMin=[]  OutMax=[]  OutDataTypeStr=double  OutputDataTypeScalingMode=double  OutDataType=fixdt(0,8)  ConRadixGroup=Best Precision: Vector-wise  OutScaling=2^-12
  Repeating Sequence Stair2 : simulink/Sources/Repeating Sequence Stair  OutValues=[0 0 1 0].'  tsamp=.01  OutMin=[]  OutMax=[]  OutDataTypeStr=double  OutputDataTypeScalingMode=double  OutDataType=fixdt(0,8)  ConRadixGroup=Best Precision: Vector-wise  OutScaling=2^-12
  Repeating Sequence Stair3 : simulink/Sources/Repeating Sequence Stair  OutValues=[0 1 0 0].'  tsamp=.01  OutMin=[]  OutMax=[]  OutDataTypeStr=double  OutputDataTypeScalingMode=double  OutDataType=fixdt(0,8)  ConRadixGroup=Best Precision: Vector-wise  OutScaling=2^-12
  Repeating Sequence Stair4 : simulink/Sources/Repeating Sequence Stair  OutValues=[1 0 0 0].'  tsamp=.01  OutMin=[]  OutMax=[]  OutDataTypeStr=double  OutputDataTypeScalingMode=double  OutDataType=fixdt(0,8)  ConRadixGroup=Best Precision: Vector-wise  OutScaling=2^-12
  Scope{7..10} (4 alike) : Scope
  Switch{2,28..30} (4 alike) : Switch  Criteria=u2 > Threshold  Threshold=110  SaturateOnIntegerOverflow=off  InputSameDT=off
  Out9 : Outport
  Out10 : Outport  Port=2
  Out11 : Outport  Port=3
  Out12 : Outport  Port=4
  Out1 : Outport  Port=5
  wires:
  Enable Stepper Pulses/1(Out1) -> Edge Detector21/1, Switch2/3
  Memory31/1 -> Out1/1
  Memory24/1 -> Add25/2
  Repeating Sequence Stair1/1 -> Enable Stepper Pulses/1(In1)
  Repeating Sequence Stair3/1 -> Enable Stepper Pulses/3(In3)
  Enable adjust = -5cm/1(Out1) -> Memory31/1
  Edge Detector24/1 -> Add27/1
  Add27/1 -> Switch30/2, Memory26/1
  Switch30/1 -> Out12/1, Scope10/1
  Switch28/1 -> Out10/1
  Constant40/1 -> Switch28/1
  Memory23/1 -> Add7/2
  Edge Detector21/1 -> Add7/1
  Enable Stepper Pulses/3(Out3) -> Edge Detector23/1, Switch29/3
  Constant37/1 -> Switch2/1
  Edge Detector22/1 -> Add25/1
  Memory26/1 -> Add27/2
  Repeating Sequence Stair4/1 -> Enable Stepper Pulses/4(In4)
  Constant41/1 -> Switch29/1
  Enable Stepper Pulses/2(Out2) -> Edge Detector22/1, Switch28/3
  Add26/1 -> Switch29/2, Memory25/1
  Memory25/1 -> Add26/2
  Edge Detector23/1 -> Add26/1
  Add7/1 -> Display5/1, Switch2/2, Memory23/1
  Enable Stepper Pulses/4(Out4) -> Edge Detector24/1, Switch30/3
  Repeating Sequence Stair2/1 -> Enable Stepper Pulses/2(In2)
  Switch29/1 -> Out11/1
  Memory27/1 -> Relational Operator4/1
  Relational Operator4/1 -> Scope9/1, Enable adjust = -5cm/Enable, Display11/1
  Add25/1 -> Switch28/2, Memory24/1
  Constant47/1 -> Enable adjust = -5cm/1(In1)
  Edge Detector25/1 -> Add28/1
  Constant42/1 -> Switch30/1
  Memory29/1 -> Add28/2
  Add28/1 -> Memory27/1, Scope8/1, Display12/1, Memory29/1
  Constant43/1 -> Relational Operator4/2
  Switch2/1 -> Out9/1, Edge Detector25/1, Scope7/1
  In1/1 -> Enable Stepper Pulses/Enable

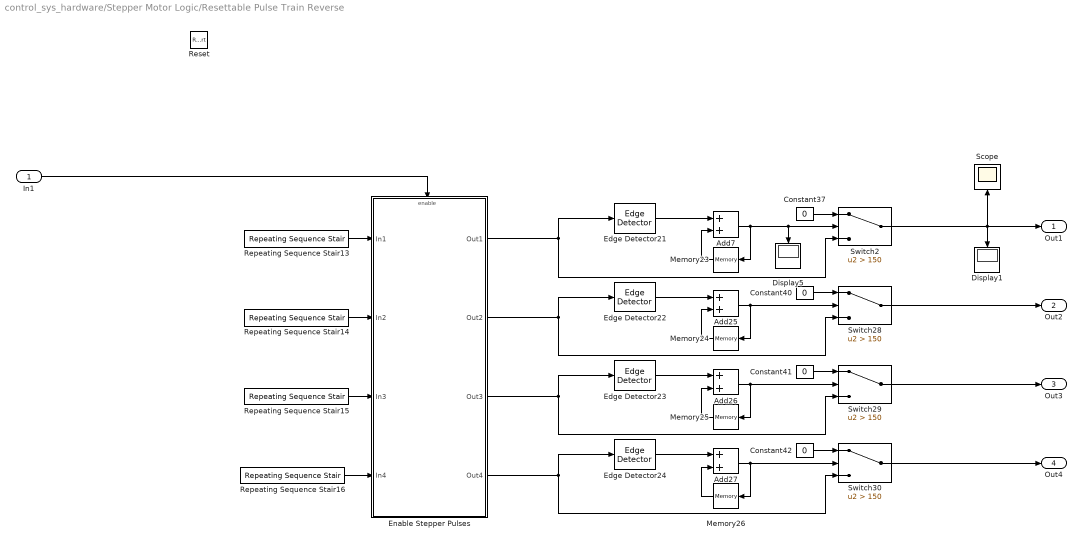
== system control_sys_hardware/Stepper Motor Logic/Resettable Pulse Train Reverse ==
  In1 : Inport
  Reset : ResetPort  DisableCoverage=on
  Add{7,25..27} (4 alike) : Sum  OutDataTypeStr=double  AccumDataTypeStr=double
  Constant{37,40..42} (4 alike) : Constant  Value=0
  Display1 : Display
  Display5 : Display
  Edge Detector{21..24} (4 alike) : spsEdgeDetectorLib/Edge Detector  model=Rising  ic=0  Ts=0
  Enable Stepper Pulses : Subsystem  TreatAsAtomicUnit=on
  Memory{23..26} (4 alike) : Memory  InheritSampleTime=on
  Repeating Sequence Stair13 : simulink/Sources/Repeating Sequence Stair  OutValues=[1 0 0 0].'  tsamp=.01  OutMin=[]  OutMax=[]  OutDataTypeStr=double  OutputDataTypeScalingMode=double  OutDataType=fixdt(0,8)  ConRadixGroup=Best Precision: Vector-wise  OutScaling=2^-12
  Repeating Sequence Stair14 : simulink/Sources/Repeating Sequence Stair  OutValues=[0 1 0 0].'  tsamp=.01  OutMin=[]  OutMax=[]  OutDataTypeStr=double  OutputDataTypeScalingMode=double  OutDataType=fixdt(0,8)  ConRadixGroup=Best Precision: Vector-wise  OutScaling=2^-12
  Repeating Sequence Stair15 : simulink/Sources/Repeating Sequence Stair  OutValues=[0 0 1 0].'  tsamp=.01  OutMin=[]  OutMax=[]  OutDataTypeStr=double  OutputDataTypeScalingMode=double  OutDataType=fixdt(0,8)  ConRadixGroup=Best Precision: Vector-wise  OutScaling=2^-12
  Repeating Sequence Stair16 : simulink/Sources/Repeating Sequence Stair  OutValues=[0 0 0 1].'  tsamp=.01  OutMin=[]  OutMax=[]  OutDataTypeStr=double  OutputDataTypeScalingMode=double  OutDataType=fixdt(0,8)  ConRadixGroup=Best Precision: Vector-wise  OutScaling=2^-12
  Scope : Scope
  Switch{2,28..30} (4 alike) : Switch  Criteria=u2 > Threshold  Threshold=150  SaturateOnIntegerOverflow=off  InputSameDT=off
  Out1 : Outport
  Out2 : Outport  Port=2
  Out3 : Outport  Port=3
  Out4 : Outport  Port=4
  wires:
  Edge Detector23/1 -> Add26/1
  In1/1 -> Enable Stepper Pulses/Enable
  Add7/1 -> Display5/1, Switch2/2, Memory23/1
  Repeating Sequence Stair13/1 -> Enable Stepper Pulses/1(In1)
  Constant42/1 -> Switch30/1
  Repeating Sequence Stair15/1 -> Enable Stepper Pulses/3(In3)
  Memory24/1 -> Add25/2
  Add25/1 -> Switch28/2, Memory24/1
  Constant41/1 -> Switch29/1
  Edge Detector21/1 -> Add7/1
  Enable Stepper Pulses/4(Out4) -> Edge Detector24/1, Switch30/3
  Memory23/1 -> Add7/2
  Constant37/1 -> Switch2/1
  Add27/1 -> Switch30/2, Memory26/1
  Enable Stepper Pulses/3(Out3) -> Edge Detector23/1, Switch29/3
  Edge Detector22/1 -> Add25/1
  Constant40/1 -> Switch28/1
  Memory26/1 -> Add27/2
  Edge Detector24/1 -> Add27/1
  Enable Stepper Pulses/2(Out2) -> Edge Detector22/1, Switch28/3
  Memory25/1 -> Add26/2
  Repeating Sequence Stair14/1 -> Enable Stepper Pulses/2(In2)
  Repeating Sequence Stair16/1 -> Enable Stepper Pulses/4(In4)
  Enable Stepper Pulses/1(Out1) -> Edge Detector21/1, Switch2/3
  Add26/1 -> Switch29/2, Memory25/1
  Switch2/1 -> Scope/1, Display1/1, Out1/1
  Switch28/1 -> Out2/1
  Switch29/1 -> Out3/1
  Switch30/1 -> Out4/1

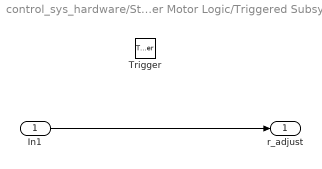
== system control_sys_hardware/Stepper Motor Logic/Triggered Subsystem ==
  In1 : Inport
  Trigger : TriggerPort  VariantControl=(inherit)
  r_adjust : Outport
  wires:
  In1/1 -> r_adjust/1

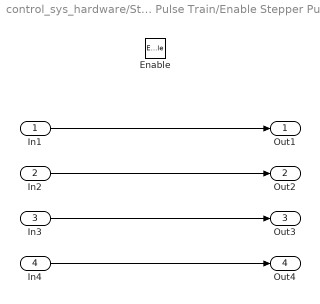
== system control_sys_hardware/Stepper Motor Logic/Resettable Pulse Train/Enable Stepper Pulses ==
  In1 : Inport
  In2 : Inport  Port=2
  In3 : Inport  Port=3
  In4 : Inport  Port=4
  Enable : EnablePort  StatesWhenEnabling=reset
  Out1 : Outport  OutputWhenDisabled=reset  InitialOutput=[0]
  Out2 : Outport  Port=2  OutputWhenDisabled=reset  InitialOutput=[0]
  Out3 : Outport  Port=3  OutputWhenDisabled=reset  InitialOutput=[0]
  Out4 : Outport  Port=4  OutputWhenDisabled=reset  InitialOutput=[0]
  wires:
  In1/1 -> Out1/1
  In2/1 -> Out2/1
  In3/1 -> Out3/1
  In4/1 -> Out4/1

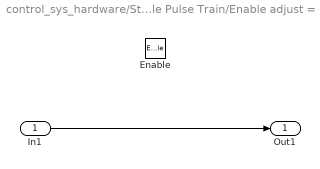
== system control_sys_hardware/Stepper Motor Logic/Resettable Pulse Train/Enable adjust = -5cm ==
  In1 : Inport
  Enable : EnablePort  StatesWhenEnabling=reset
  Out1 : Outport  SampleTime=.01  OutputWhenDisabled=reset  InitialOutput=[0]
  wires:
  In1/1 -> Out1/1

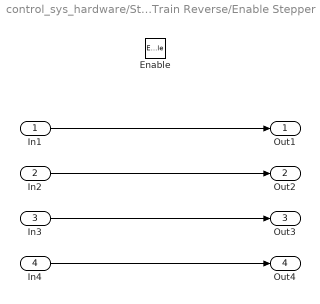
== system control_sys_hardware/Stepper Motor Logic/Resettable Pulse Train Reverse/Enable Stepper Pulses ==
  In1 : Inport
  In2 : Inport  Port=2
  In3 : Inport  Port=3
  In4 : Inport  Port=4
  Enable : EnablePort  StatesWhenEnabling=reset
  Out1 : Outport  OutputWhenDisabled=reset  InitialOutput=[0]
  Out2 : Outport  Port=2  OutputWhenDisabled=reset  InitialOutput=[0]
  Out3 : Outport  Port=3  OutputWhenDisabled=reset  InitialOutput=[0]
  Out4 : Outport  Port=4  OutputWhenDisabled=reset  InitialOutput=[0]
  wires:
  In1/1 -> Out1/1
  In2/1 -> Out2/1
  In3/1 -> Out3/1
  In4/1 -> Out4/1

== matlab function control_sys_hardware/Gain Schedule ==
  data: theta input; K output
function K = compute_gains(theta)
    if theta < pi/4
        K = [14.1421, 4.8365, 0.7439, -0.0100   -0.0024   -0.0000    0.0000    0.0000    0.0000
   -0.0086   -0.0048   -0.0002  100.4219   47.2763    2.8226   -0.0061   -0.0001   -0.0000
    0.0000    0.0000    0.0000    0.0005   -0.0004   -0.0000  447.2136 -502.7700   11.8456]; %@ 0 rad
    else
        K = [14.1421, 4.8365, 0.7439, -0.0040, -0.0009, -0.0000, 0.0000, 0.0000, 0.0000;
            -0.0034, -0.0019, -0.0001, 100.4219, 47.2825, 2.8225, 0.0011, 0.0003, 0.0000;
            0.0000, 0.0000, 0.0000, 0.0041, 0.0006, 0.0000, 632.4555, -514.8569, 11.9155]; %@ pi/2 rad
    end
end

== matlab function control_sys_hardware/MATLAB Function ==
  data: i input; phi_ref output; positions input; theta_ref output; r_ref output
function [phi_ref, theta_ref, r_ref] = getNextPosition(i,positions)
for c = 1:length(positions(1,:))
    phi_ref = positions(1,i);
    theta_ref = positions(2,i);
    r_ref = positions(3,i);
end
